simulink model "MPM_v3_16b"  (R2016b)
settings: Solver=ode4  StartTime=0.0  StopTime=5  RelTol=1e-3
settings Model: SimulationMode=accelerator  Creator=HYJ  LastModifiedBy=HYJ
settings SFSimCC: SimUseLocalCustomCode=on
settings RTWCC: RTWUseLocalCustomCode=on

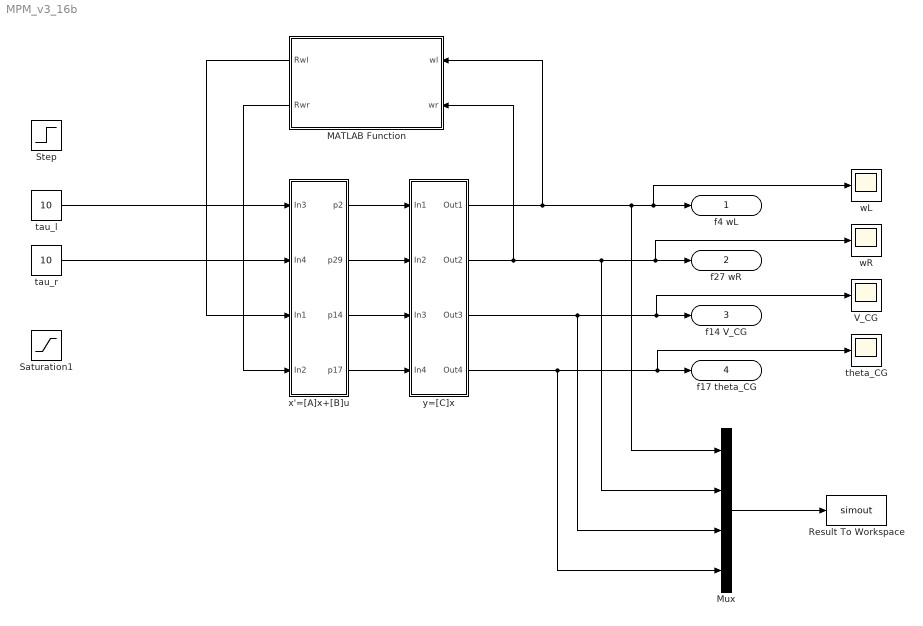
== system MPM_v3_16b ==
  MATLAB Function : MATLAB Function  TreatAsAtomicUnit=on
  Mux : Mux
  Result To Workspace : ToWorkspace  VariableName=simout  SaveFormat=Timeseries  SampleTime=-1
  Saturation1 : Saturate  UpperLimit=30  LowerLimit=-30
  Step : Step  Time=3  After=4  SampleTime=0
  V_CG : Scope
  tau_l : Constant  Value=10
  tau_r : Constant  Value=10
  theta_CG : Scope
  wL : Scope
  wR : Scope
  x'=[A]x+[B]u : Subsystem  mask{Rg=0.006, Jw=0.005, Cwc=0.005, Rwc=0.005, Cw=0.021, Rw=12, Jt=64, Mt=100, r=0.3}
  y=[C]x : Subsystem  mask{Jw=0.005, Mt=100, Jt=64}
  f4 wL : Outport
  f27 wR : Outport  Port=2
  f14 V_CG : Outport  Port=3
  f17 theta_CG : Outport  Port=4
  wires:
  y=[C]x/2(Out2) -> Mux/2, wR/1, f27 wR/1, MATLAB Function/2(wr)
  y=[C]x/1(Out1) -> MATLAB Function/1(wl), Mux/1, wL/1, f4 wL/1
  x'=[A]x+[B]u/1(p2) -> y=[C]x/1(In1)
  x'=[A]x+[B]u/2(p29) -> y=[C]x/2(In2)
  x'=[A]x+[B]u/3(p14) -> y=[C]x/3(In3)
  x'=[A]x+[B]u/4(p17) -> y=[C]x/4(In4)
  Mux/1 -> Result To Workspace/1
  MATLAB Function/1(Rwl) -> x'=[A]x+[B]u/3(In1)
  MATLAB Function/2(Rwr) -> x'=[A]x+[B]u/4(In2)
  y=[C]x/3(Out3) -> Mux/3, V_CG/1, f14 V_CG/1
  y=[C]x/4(Out4) -> Mux/4, theta_CG/1, f17 theta_CG/1
  tau_l/1 -> x'=[A]x+[B]u/1(In3)
  tau_r/1 -> x'=[A]x+[B]u/2(In4)

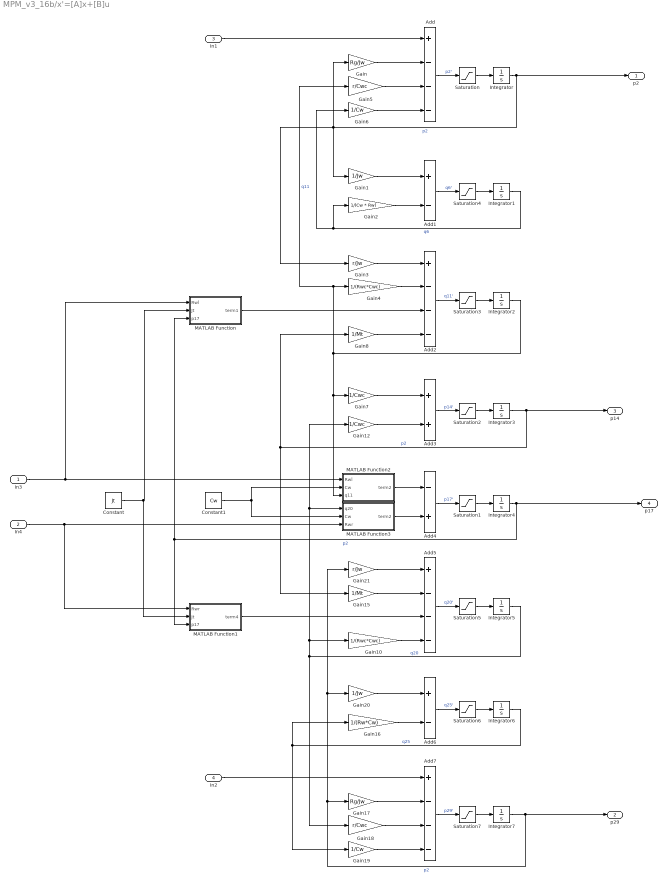
== system MPM_v3_16b/x'=[A]x+[B]u ==
  In3 : Inport
  In4 : Inport  Port=2
  In1 : Inport  Port=3
  In2 : Inport  Port=4
  Add{,2,5,7} (4 alike) : Sum  Inputs=+---
  Add1 : Sum  Inputs=+-
  Add3 : Sum
  Add4 : Sum  Inputs=-+
  Add6 : Sum  Inputs=+-
  Constant : Constant  Value=Jt
  Constant1 : Constant  Value=Cw
  Gain : Gain  Gain=Rg/Jw
  Gain1 : Gain  Gain=1/Jw
  Gain10 : Gain  Gain=1/(Rwc*Cwc)
  Gain12 : Gain  Gain=1/Cwc
  Gain15 : Gain  Gain=1/Mt
  Gain16 : Gain  Gain=1/(Rw*Cw)
  Gain17 : Gain  Gain=Rg/Jw
  Gain18 : Gain  Gain=r/Cwc
  Gain19 : Gain  Gain=1/Cw
  Gain2 : Gain  Gain=1/(Cw * Rw)
  Gain20 : Gain  Gain=1/Jw
  Gain21 : Gain  Gain=r/Jw
  Gain3 : Gain  Gain=r/Jw
  Gain4 : Gain  Gain=1/(Rwc*Cwc)
  Gain5 : Gain  Gain=r/Cwc
  Gain6 : Gain  Gain=1/Cw
  Gain7 : Gain  Gain=1/Cwc
  Gain8 : Gain  Gain=1/Mt
  Integrator{,1..3,5..7} (7 alike) : Integrator
  Integrator4 : Integrator  InitialCondition=0.001
  MATLAB Function : MATLAB Function  TreatAsAtomicUnit=on
  MATLAB Function1 : MATLAB Function  TreatAsAtomicUnit=on
  MATLAB Function2 : MATLAB Function  TreatAsAtomicUnit=on
  MATLAB Function3 : MATLAB Function  TreatAsAtomicUnit=on
  Saturation{,2..7} (7 alike) : Saturate  UpperLimit=100  LowerLimit=-100
  Saturation1 : Saturate  UpperLimit=50  LowerLimit=-50
  p2 : Outport
  p29 : Outport  Port=2
  p14 : Outport  Port=3
  p17 : Outport  Port=4
  wires:
  Add3/1 -> Saturation2/1  "p14'"
  Gain/1 -> Add/2
  In2/1 -> Add7/1
  Add7/1 -> Saturation7/1  "p29'"
  Integrator/1 -> p2/1, Gain3/1, Gain1/1, Gain/1  "p2"
  Integrator2/1 -> Gain4/1, Gain5/1, MATLAB Function2/3(q11), Gain7/1  "q11"
  Add2/1 -> Saturation3/1  "q11'"
  Gain19/1 -> Add7/4
  Gain1/1 -> Add1/1
  Gain10/1 -> Add5/4
  Integrator1/1 -> Gain6/1, Gain2/1  "q6"
  Gain17/1 -> Add7/2
  Integrator5/1 -> Gain10/1, Gain12/1, MATLAB Function3/1(q20), Gain18/1  "q20"
  Gain5/1 -> Add/3
  Add1/1 -> Saturation4/1  "q6'"
  Gain20/1 -> Add6/1
  Gain6/1 -> Add/4
  Add4/1 -> Saturation1/1  "p17'"
  Gain16/1 -> Add6/2
  Gain18/1 -> Add7/3
  MATLAB Function1/1(term4) -> Add5/3
  Gain2/1 -> Add1/2
  MATLAB Function2/1(term2) -> Add4/1
  Gain15/1 -> Add5/2
  Gain8/1 -> Add2/4
  Integrator6/1 -> Gain19/1, Gain16/1  "q25"
  Gain3/1 -> Add2/1
  Gain4/1 -> Add2/2
  Add5/1 -> Saturation5/1  "q20'"
  Gain21/1 -> Add5/1
  Gain7/1 -> Add3/1
  Gain12/1 -> Add3/2
  In1/1 -> Add/1
  Add6/1 -> Saturation6/1  "q25'"
  Integrator3/1 -> p14/1, Gain8/1, Gain15/1  "p2"
  Integrator7/1 -> p29/1, Gain21/1, Gain20/1, Gain17/1  "p2"
  Integrator4/1 -> p17/1, MATLAB Function1/3(p17), MATLAB Function/3(p17)  "p2"
  In3/1 -> MATLAB Function/1(Rwl), MATLAB Function2/1(Rwl)
  In4/1 -> MATLAB Function3/3(Rwr), MATLAB Function1/1(Rwr)
  MATLAB Function/1(term1) -> Add2/3
  Constant/1 -> MATLAB Function1/2(Jt), MATLAB Function/2(Jt)
  Constant1/1 -> MATLAB Function2/2(Cw), MATLAB Function3/2(Cw)
  MATLAB Function3/1(term2) -> Add4/2
  Add/1 -> Saturation/1  "p2'"
  Saturation/1 -> Integrator/1
  Saturation1/1 -> Integrator4/1
  Saturation2/1 -> Integrator3/1
  Saturation3/1 -> Integrator2/1
  Saturation4/1 -> Integrator1/1
  Saturation5/1 -> Integrator5/1
  Saturation6/1 -> Integrator6/1
  Saturation7/1 -> Integrator7/1

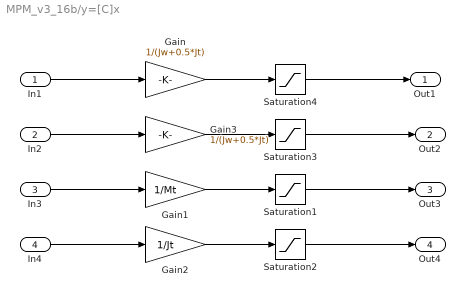
== system MPM_v3_16b/y=[C]x ==
  In1 : Inport
  In2 : Inport  Port=2
  In3 : Inport  Port=3
  In4 : Inport  Port=4
  Gain : Gain  Gain=1/(Jw+0.5*Jt)
  Gain1 : Gain  Gain=1/Mt
  Gain2 : Gain  Gain=1/Jt
  Gain3 : Gain  Gain=1/(Jw+0.5*Jt)
  Saturation1 : Saturate  UpperLimit=10  LowerLimit=-10
  Saturation2 : Saturate  UpperLimit=10  LowerLimit=-10
  Saturation3 : Saturate  UpperLimit=50  LowerLimit=-30  ZeroCross=off
  Saturation4 : Saturate  UpperLimit=100  LowerLimit=-30  ZeroCross=off
  Out1 : Outport
  Out2 : Outport  Port=2
  Out3 : Outport  Port=3
  Out4 : Outport  Port=4
  wires:
  Gain3/1 -> Saturation3/1
  In3/1 -> Gain1/1
  Gain2/1 -> Saturation2/1
  Gain/1 -> Saturation4/1
  Gain1/1 -> Saturation1/1
  In4/1 -> Gain2/1
  In2/1 -> Gain3/1
  In1/1 -> Gain/1
  Saturation1/1 -> Out3/1
  Saturation2/1 -> Out4/1
  Saturation3/1 -> Out2/1
  Saturation4/1 -> Out1/1

== matlab function MPM_v3_16b/x'=[A]x+[B]u/MATLAB Function ==
  data: Rwl input; term1 output; Jt input; p17 input
function term1 = dyna_input1(Rwl, Jt, p17)
if Rwl == Inf
    term1 = 0;
else
    term1 = p17/(Jt*Rwl);
end
end

== matlab function MPM_v3_16b/MATLAB Function ==
  data: wl input; Rwl output; Rwr output; wr input
function [Rwl, Rwr] = rotation_radius_compution(wl, wr)
% 输入两后轮各自角速度，输出两轮围绕瞬心的曲率半径
Lw = 0.8; % 轮椅左右轮宽度
if wl > wr
    Rwl = (Lw * max(wl, wr))/abs(wl - wr);
    Rwr = (Lw * min(wl, wr))/abs(wl - wr);
elseif wr > wl
    Rwr = (Lw * max(wl, wr))/abs(wl - wr);
    Rwl = (Lw * min(wl, wr))/abs(wl - wr);
else
    Rwl = Inf; % 1e15
    Rwr = Inf; % 1e15
end
end

== matlab function MPM_v3_16b/x'=[A]x+[B]u/MATLAB Function1 ==
  data: Rwr input; term4 output; Jt input; p17 input
function term4 = dyna_input4(Rwr, Jt, p17)
if Rwr == Inf
    term4 = 0;
else
    term4 = p17/(Jt*Rwr);
end
end

== matlab function MPM_v3_16b/x'=[A]x+[B]u/MATLAB Function2 ==
  data: Rwl input; term2 output; Cw input; q11 input
function term2 = dyna_input2(Rwl, Cw, q11)
if Rwl == Inf
    term2 = 0;
else
    term2 = q11/(Cw*Rwl);
end
end

== matlab function MPM_v3_16b/x'=[A]x+[B]u/MATLAB Function3 ==
  data: q20 input; Cw input; Rwr input; term2 output
function term2 = dyna_input2(q20, Cw, Rwr)
if Rwr == Inf
    term2 = 0;
else
    term2 = q20/(Cw*Rwr);
end
end
